simulink model "P5_Manipuladores"  (R2023b)
settings: Solver=VariableStepAuto  StartTime=0.0  StopTime=10  RelTol=1e-3
undefined symbols (not defined in the file): Cf, K, Kd, KF, KI, Kp, Md, xe_inicial
settings Model: Creator=manu_  LastModifiedBy=manu_

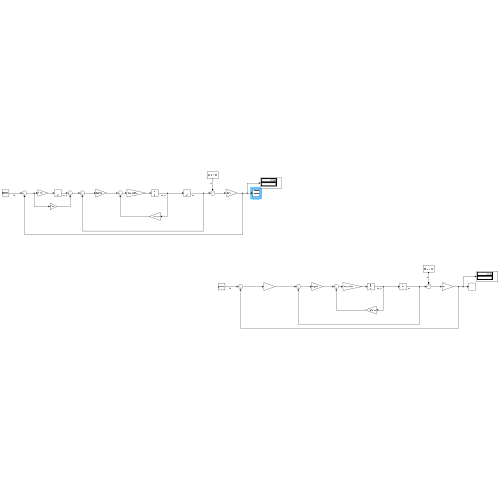
[thumbnail: Simulink's stored preview of the top-level diagram]
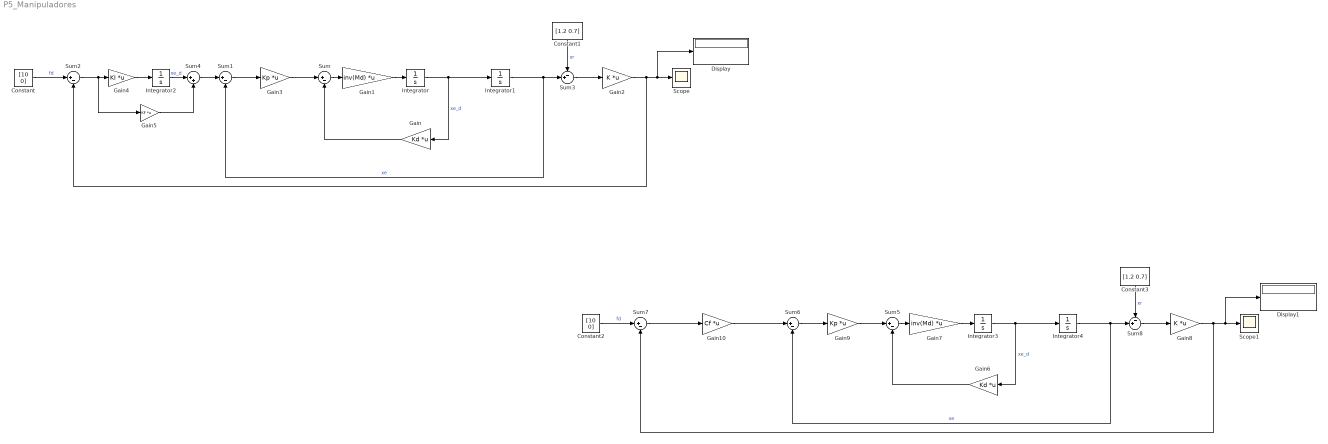
== system P5_Manipuladores ==
  Constant : Constant  Value=[10 0]
  Constant1 : Constant  Value=[1.2 0.7]
  Constant2 : Constant  Value=[10 0]
  Constant3 : Constant  Value=[1.2 0.7]
  Display : Display
  Display1 : Display
  Gain : Gain  Gain=Kd  Multiplication=Matrix(K*u)
  Gain1 : Gain  Gain=inv(Md)  Multiplication=Matrix(K*u)
  Gain10 : Gain  Gain=Cf  Multiplication=Matrix(K*u)
  Gain2 : Gain  Gain=K  Multiplication=Matrix(K*u)
  Gain3 : Gain  Gain=Kp  Multiplication=Matrix(K*u)
  Gain4 : Gain  Gain=KI  Multiplication=Matrix(K*u)
  Gain5 : Gain  Gain=KF  Multiplication=Matrix(K*u)
  Gain6 : Gain  Gain=Kd  Multiplication=Matrix(K*u)
  Gain7 : Gain  Gain=inv(Md)  Multiplication=Matrix(K*u)
  Gain8 : Gain  Gain=K  Multiplication=Matrix(K*u)
  Gain9 : Gain  Gain=Kp  Multiplication=Matrix(K*u)
  Integrator{,1..4} (5 alike) : Integrator  InitialCondition=xe_inicial
  Scope : Scope
  Scope1 : Scope
  Sum{,1..2,5..7} (6 alike) : Sum  Inputs=|+-
  Sum3 : Sum  Inputs=-+|
  Sum4 : Sum  Inputs=|++
  Sum8 : Sum  Inputs=-+|
  wires:
  Integrator/1 -> Gain/1, Integrator1/1  "xe_d"
  Sum/1 -> Gain1/1
  Gain1/1 -> Integrator/1
  Integrator1/1 -> Sum3/2, Sum1/2  "xe"
  Constant1/1 -> Sum3/1  "xr"
  Constant/1 -> Sum2/1  "fd"
  Sum1/1 -> Gain3/1
  Gain3/1 -> Sum/1
  Gain/1 -> Sum/2
  Sum3/1 -> Gain2/1
  Gain2/1 -> Sum2/2, Display/1, Scope/1
  Sum2/1 -> Gain5/1, Gain4/1
  Gain4/1 -> Integrator2/1
  Sum4/1 -> Sum1/1
  Integrator2/1 -> Sum4/1  "xe_d"
  Gain5/1 -> Sum4/2
  Sum5/1 -> Gain7/1
  Integrator3/1 -> Gain6/1, Integrator4/1  "xe_d"
  Constant3/1 -> Sum8/1  "xr"
  Sum8/1 -> Gain8/1
  Constant2/1 -> Sum7/1  "fd"
  Gain8/1 -> Sum7/2, Display1/1, Scope1/1
  Gain7/1 -> Integrator3/1
  Sum6/1 -> Gain9/1
  Gain9/1 -> Sum5/1
  Gain6/1 -> Sum5/2
  Integrator4/1 -> Sum8/2, Sum6/2  "xe"
  Sum7/1 -> Gain10/1
  Gain10/1 -> Sum6/1
